simulink model "pend_MN_sim"  (R2013a)
settings: Solver=ode4  StartTime=0.0  StopTime=max(t)  FixedStep=h  RelTol=1e-3
values from neighbouring files (symbols this model uses):
  g = 9.81    [RotatedPendulumParams.m]    (also in ident_pend.m; rotary_ip_lq.m)
  l2 = 20e-2    (= 0.2)    [RotatedPendulumParams.m]    (also in ident_pend.m = 0.071; rotary_ip_lq.m = 0.071)
  m2 = 40e-3    (= 0.04)    [RotatedPendulumParams.m]    (also in ident_pend.m = 0.004; rotary_ip_lq.m = 0.004)
  Tf2 = 0.025    [ident_pend.m]    (also in rotary_ip_lq.m = 0.06)
libraries: cstblocks x3
settings Model: Creator=kawata  LastModifiedBy=kawata
settings DataIOCC: SignalLoggingSaveFormat=ModelDataLogs
settings OptimizationCC: ExpressionDepthLimit=2147483647
settings DebuggingCC: FcnCallInpInsideContextMsg=UseLocalSettings
settings GRTTargetCC: CombineOutputUpdateFcns=off  GRTInterface=on

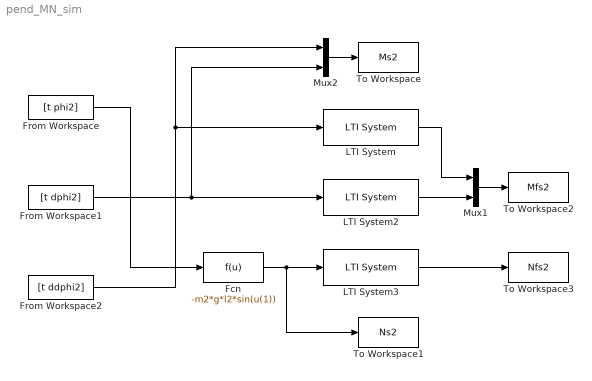
== system pend_MN_sim ==
  Fcn : Fcn  Expr=-m2*g*l2*sin(u(1))
  From Workspace : FromWorkspace  VariableName=[t phi2]  SampleTime=0
  From Workspace1 : FromWorkspace  VariableName=[t dphi2]  SampleTime=0
  From Workspace2 : FromWorkspace  VariableName=[t ddphi2]  SampleTime=0
  LTI System : cstblocks/LTI System  sys=tf(1,[Tf2 1])^3  IC=[]
  LTI System2 : cstblocks/LTI System  sys=tf(1,[Tf2 1])^3  IC=[]
  LTI System3 : cstblocks/LTI System  sys=tf(1,[Tf2 1])^3  IC=[]
  Mux1 : Mux  Inputs=2
  Mux2 : Mux  Inputs=2
  To Workspace : ToWorkspace  VariableName=Ms2  SampleTime=-1
  To Workspace1 : ToWorkspace  VariableName=Ns2  SampleTime=-1
  To Workspace2 : ToWorkspace  VariableName=Mfs2  SampleTime=-1
  To Workspace3 : ToWorkspace  VariableName=Nfs2  SampleTime=-1
  wires:
  Mux1/1 -> To Workspace2/1
  LTI System/1 -> Mux1/1
  LTI System2/1 -> Mux1/2
  From Workspace1/1 -> Mux2/2, LTI System2/1
  Fcn/1 -> To Workspace1/1, LTI System3/1
  LTI System3/1 -> To Workspace3/1
  From Workspace/1 -> Fcn/1
  From Workspace2/1 -> Mux2/1, LTI System/1
  Mux2/1 -> To Workspace/1
